simulink library "fsw_lib"  (R2016b)
settings: Solver=ode45  StartTime=0.0  StopTime=10.0  RelTol=1e-3  EnableMultiTasking=on
undefined symbols (not defined in the file or in its folder): att_ki, att_kp, bus_ctl_input_msg_ic, cmd_state_a, cmd_state_b, ctl_mode_cmd, current_time_nsec, current_time_sec, est_confidence, est_omega_B_ISS_B, est_P_B_ISS_ISS, est_quat_ISS2B, est_V_B_ISS_ISS, inertia_matrix, mass, omega_kd, pos_ki, pos_kp, speed_gain_cmd, tun_debug_ctl_use_truth, vel_kd
libraries: ctl_controller x1, est_estimator_lib_wState_lib x1, fam_force_allocation_module_lib x1
settings Model: Creator=jfusco1  LastModifiedBy=jfusco1
settings DataIOCC: LimitDataPoints=on  SaveFormat=Array
settings OptimizationCC: LifeSpan=inf
settings DebuggingCC: SolverPrmCheckMsg=warning  AllowSymbolicDim=off  SFUnexpectedBacktrackingDiag=warning  SFNoUnconditionalDefaultTransitionDiag=warning  SFExecutionAtInitializationDiag=none
settings HardwareCC: ProdBitPerPointer=32  ProdBitPerSizeT=32  ProdBitPerPtrDiffT=32  ProdLargestAtomicFloat=None  ProdIntDivRoundTo=Undefined  ProdEndianess=Unspecified  ProdWordSize=32  ProdHWDeviceType=32-bit Generic
settings ModelReferenceCC: PropagateSignalLabelsOutOfModel=off
settings GRTTargetCC: TargetLangStandard=C89/C90 (ANSI)  GeneratePreprocessorConditionals=Disable all
settings ConfigComp: CovMetricSettings=dw  CovHtmlReporting=on  CovSaveCumulativeToWorkspaceVar=on  CovSaveSingleToWorkspaceVar=on  CovExternalEMLEnable=off  CovSFcnEnable=off

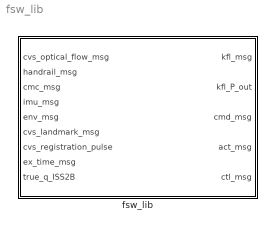
== system fsw_lib ==
  fsw_lib : Subsystem

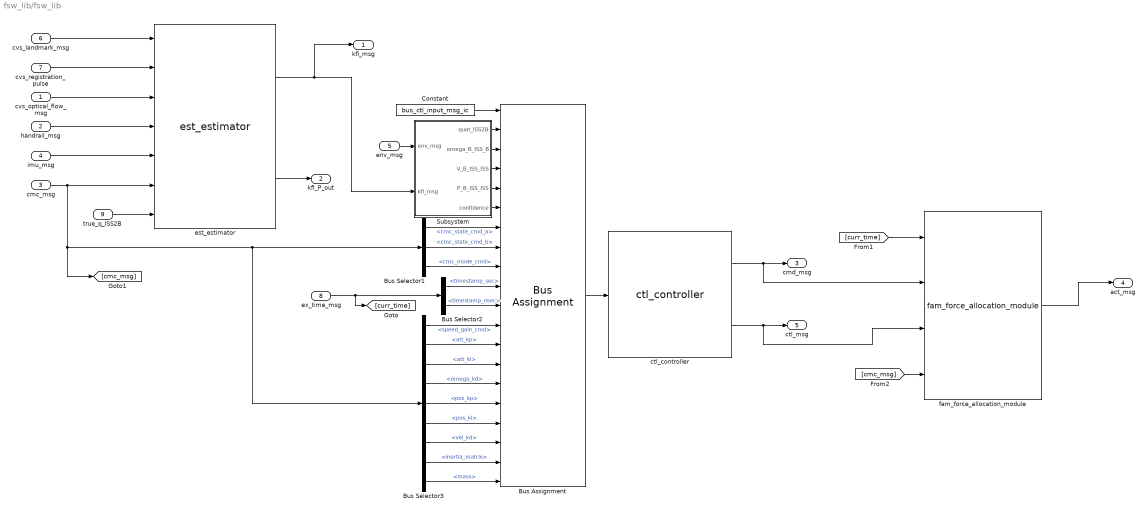
== system fsw_lib/fsw_lib ==
  cvs_optical_flow_msg : Inport  OutDataTypeStr=Bus: cvs_optical_flow_msg
  handrail_msg : Inport  Port=2
  cmc_msg : Inport  Port=3  OutDataTypeStr=Bus: cmc_msg
  imu_msg : Inport  Port=4  OutDataTypeStr=Bus: imu_msg
  env_msg : Inport  Port=5  OutDataTypeStr=Bus: env_msg
  cvs_landmark_msg : Inport  Port=6  OutDataTypeStr=Bus: cvs_landmark_msg
  cvs_registration_pulse : Inport  Port=7  OutDataTypeStr=Bus: cvs_registration_pulse
  ex_time_msg : Inport  Port=8  OutDataTypeStr=Bus: ex_time_msg
  true_q_ISS2B : Inport  Port=9
  Bus Assignment : BusAssignment  AssignedSignals=est_quat_ISS2B,est_omega_B_ISS_B,est_V_B_ISS_ISS,est_P_B_ISS_ISS,est_confidence,cmd_state_a,cmd_state_b,ctl_mode_cmd,current_time_sec,current_time_nsec,speed_gain_cmd,att_kp,att_ki,omega_kd,pos_kp,pos_ki,vel_kd,inertia_matrix,mass
  Bus Selector1 : BusSelector  OutputSignals=cmc_state_cmd_a,cmc_state_cmd_b,cmc_mode_cmd
  Bus Selector2 : BusSelector  OutputSignals=timestamp_sec,timestamp_nsec
  Bus Selector3 : BusSelector  OutputSignals=speed_gain_cmd,att_kp,att_ki,omega_kd,pos_kp,pos_ki,vel_kd,inertia_matrix,mass
  Constant : Constant  Value=bus_ctl_input_msg_ic  OutDataTypeStr=Bus: ctl_input_msg
  Subsystem : Subsystem
  ctl_controller : ctl_controller/ctl_controller
  est_estimator : est_estimator_lib_wState_lib/est_estimator
  fam_force_allocation_module : fam_force_allocation_module_lib/fam_force_allocation_module
  kfl_msg : Outport  OutDataTypeStr=Bus: kfl_msg
  kfl_P_out : Outport  Port=2
  cmd_msg : Outport  Port=3  OutDataTypeStr=Bus: cmd_msg
  act_msg : Outport  Port=4
  ctl_msg : Outport  Port=5
  wires:
  handrail_msg/1 -> est_estimator/4
  fam_force_allocation_module/1 -> act_msg/1
  [curr_time] -> fam_force_allocation_module/1
  cmc_msg/1 -> [cmc_msg], Bus Selector1/1, Bus Selector3/1, est_estimator/6
  est_estimator/1 -> Subsystem/2(kfl_msg), kfl_msg/1
  cvs_landmark_msg/1 -> est_estimator/1
  cvs_optical_flow_msg/1 -> est_estimator/3
  imu_msg/1 -> est_estimator/5
  cvs_registration_pulse/1 -> est_estimator/2
  est_estimator/2 -> kfl_P_out/1
  ctl_controller/1 -> fam_force_allocation_module/2, cmd_msg/1
  ctl_controller/2 -> fam_force_allocation_module/3, ctl_msg/1
  true_q_ISS2B/1 -> est_estimator/7
  [cmc_msg] -> fam_force_allocation_module/4
  Constant/1 -> Bus Assignment/1
  Bus Assignment/1 -> ctl_controller/1
  Subsystem/2(omega_B_ISS_B) -> Bus Assignment/3
  Subsystem/3(V_B_ISS_ISS) -> Bus Assignment/4
  Subsystem/1(quat_ISS2B) -> Bus Assignment/2
  Subsystem/4(P_B_ISS_ISS) -> Bus Assignment/5
  Subsystem/5(confidence) -> Bus Assignment/6
  Bus Selector1/1 -> Bus Assignment/7  "<cmc_state_cmd_a>"
  Bus Selector1/2 -> Bus Assignment/8  "<cmc_state_cmd_b>"
  Bus Selector1/3 -> Bus Assignment/9  "<cmc_mode_cmd>"
  ex_time_msg/1 -> [curr_time], Bus Selector2/1
  Bus Selector2/1 -> Bus Assignment/10  "<timestamp_sec>"
  Bus Selector2/2 -> Bus Assignment/11  "<timestamp_nsec>"
  Bus Selector3/1 -> Bus Assignment/12  "<speed_gain_cmd>"
  Bus Selector3/2 -> Bus Assignment/13  "<att_kp>"
  Bus Selector3/3 -> Bus Assignment/14  "<att_ki>"
  Bus Selector3/4 -> Bus Assignment/15  "<omega_kd>"
  Bus Selector3/5 -> Bus Assignment/16  "<pos_kp>"
  Bus Selector3/6 -> Bus Assignment/17  "<pos_ki>"
  Bus Selector3/7 -> Bus Assignment/18  "<vel_kd>"
  Bus Selector3/8 -> Bus Assignment/19  "<inertia_matrix>"
  Bus Selector3/9 -> Bus Assignment/20  "<mass>"
  env_msg/1 -> Subsystem/1(env_msg)

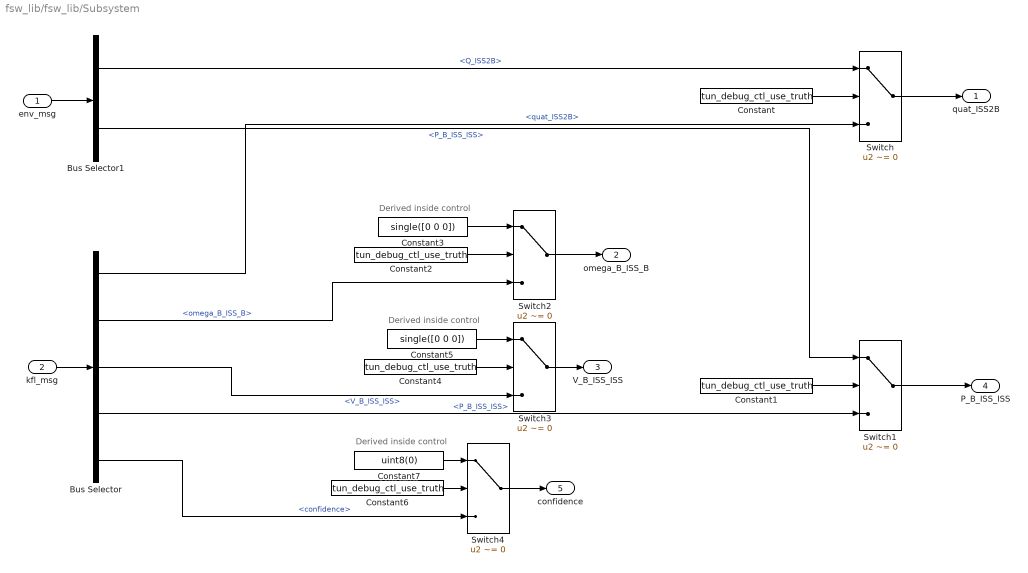
== system fsw_lib/fsw_lib/Subsystem ==
  note: Derived inside control
  note: Derived inside control
  note: Derived inside control
  env_msg : Inport  OutDataTypeStr=Bus: env_msg
  kfl_msg : Inport  Port=2  OutDataTypeStr=Bus: kfl_msg
  Bus Selector : BusSelector  OutputSignals=quat_ISS2B,omega_B_ISS_B,V_B_ISS_ISS,P_B_ISS_ISS,confidence
  Bus Selector1 : BusSelector  OutputSignals=Q_ISS2B,P_B_ISS_ISS
  Constant{,1..2,4,6} (5 alike) : Constant  Value=tun_debug_ctl_use_truth
  Constant3 : Constant  Value=single([0 0 0])
  Constant5 : Constant  Value=single([0 0 0])
  Constant7 : Constant  Value=uint8(0)
  Switch{,1..4} (5 alike) : Switch  Criteria=u2 ~= 0
  quat_ISS2B : Outport
  omega_B_ISS_B : Outport  Port=2
  V_B_ISS_ISS : Outport  Port=3
  P_B_ISS_ISS : Outport  Port=4
  confidence : Outport  Port=5
  wires:
  Constant/1 -> Switch/2
  kfl_msg/1 -> Bus Selector/1
  env_msg/1 -> Bus Selector1/1
  Bus Selector1/1 -> Switch/1  "<Q_ISS2B>"
  Switch/1 -> quat_ISS2B/1
  Bus Selector/1 -> Switch/3  "<quat_ISS2B>"
  Constant1/1 -> Switch1/2
  Bus Selector1/2 -> Switch1/1  "<P_B_ISS_ISS>"
  Bus Selector/4 -> Switch1/3  "<P_B_ISS_ISS>"
  Switch1/1 -> P_B_ISS_ISS/1
  Constant2/1 -> Switch2/2
  Bus Selector/2 -> Switch2/3  "<omega_B_ISS_B>"
  Constant3/1 -> Switch2/1
  Switch2/1 -> omega_B_ISS_B/1
  Bus Selector/3 -> Switch3/3  "<V_B_ISS_ISS>"
  Constant4/1 -> Switch3/2
  Constant5/1 -> Switch3/1
  Switch3/1 -> V_B_ISS_ISS/1
  Constant6/1 -> Switch4/2
  Bus Selector/5 -> Switch4/3  "<confidence>"
  Switch4/1 -> confidence/1
  Constant7/1 -> Switch4/1
